simulink library "AUVLib"  (R2025b)
settings: Solver=VariableStepAuto  StartTime=0.0  StopTime=10.0  RelTol=1e-3
undefined symbols (not defined in the file): AUV, waterDensity
libraries: asbAUVlib x2, matrix_library x1, aerolibadyn x1, aerolibasang x1
settings Model: Creator=abshanka  LastModifiedBy=ubuntu

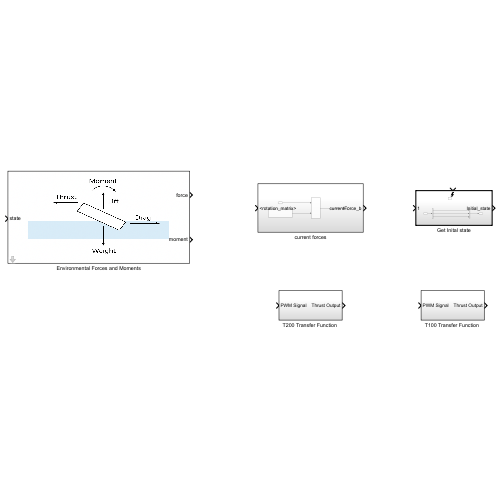
[thumbnail: Simulink's stored preview of the top-level diagram]
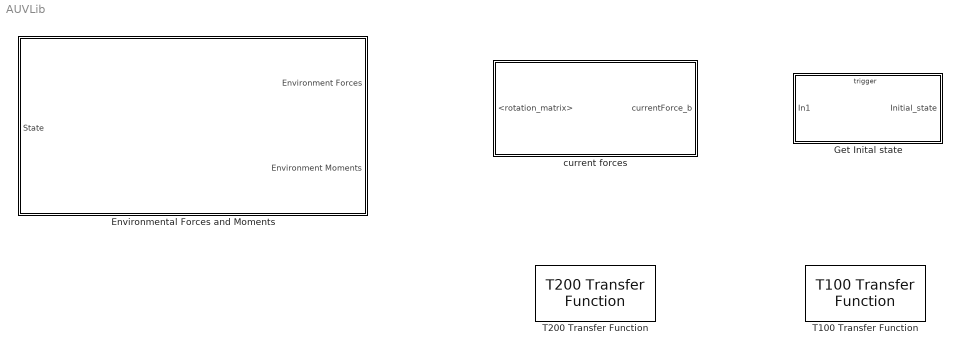
== system AUVLib ==
  Environmental Forces and Moments : Subsystem  mask{V=0.2056, h=AUV.Body.hulldiameter, mass=AUV.Body.mass, CoB=[0; 0; 0], Hy=Simple, ang_coeff=diag([ 10, 80,  82]), quad_coeff=diag([ 5,  32,  680]), lin_coeff=diag([ 3,  22,  220]), ang_coeff_c=diag([ 10, 80,  82]), alphaR=0, betaR=0, CX=0, CY=0, CZ=0, CMK=0, CMM=0, CMN=0, inputAxes=Body, cbar=1, b=1, S=1}
      mask prompts: V "Volume of AUV (m^3)"; h "Heigh (or diameter) of AUV (m)"; mass "Mass of AUV (kg)"; CoB "CoB (relative to CoM)"; Hy "Choose Hydrodynamics Simulation"; ang_coeff "Angular Damping coefficient"; quad_coeff "Quadratic drag coefficient"; lin_coeff "Linear drag coefficient"; ang_coeff_c "Angular Damping coefficient"; alphaR "Alpha Range"; betaR "Beta Range"; CX "Axial force coeff (CX)"; CY "Side force coeff (CY)"; CZ "Normal force coeff (CZ)"; CMK "Rolling moment coeff"; CMM "Pitching moment coeff"; CMN "Yawing moment coeff"; inputAxes "aeroblks:aeroblkadyn:blockAerodynamicForcesandMomentsParamInputaxes"; cbar "Length (m)"; b "Span (m)"; S "Ref Area (m^2)"
      mask TypeOptions V: Hydrostatics/volume displaced (m^3)/Value
      mask TypeOptions h: Hydrostatics/height/Value
      mask TypeOptions mass: Hydrostatics/Mass (Kg)/Value
      mask TypeOptions CoB: Hydrostatics/CoB (relative to CoM)(m)/Value
      mask TypeOptions inputAxes:
      | Variant Subsystem/Hydrodynamics_complex/Aerodynamic
      | Forces and Moments /inputAxes
      mask TypeOptions cbar:
      | Variant Subsystem/Hydrodynamics_complex/Aerodynamic
      | Forces and Moments /cbar
      mask TypeOptions b:
      | Variant Subsystem/Hydrodynamics_complex/Aerodynamic
      | Forces and Moments /b
      mask TypeOptions S:
      | Variant Subsystem/Hydrodynamics_complex/Aerodynamic
      | Forces and Moments /S
      mask DialogControl AUV_general Prompt: AUV Parameters (General)
      mask DialogControl AUV_hydro Prompt: AUV Hydrodynamics
      mask DialogControl Container5 Prompt: Simple Hydrodynamic Coeffs
      mask DialogControl Container6 Prompt: Complex Hydroynamics Coeffs
      mask DialogControl inputAxes Prompt: Input axes:
      mask Display:
      | image('force_moment.png');
      | port_label('output', 1, 'force');
      | port_label('output', 2, 'moment');
      | port_label('input', 1, 'state');
  Get Inital state : Subsystem
  "T100 Transfer Function " : asbAUVlib/T100 Transfer Function  SystemSampleTime=-1  VariantActivationTime=update diagram  EmptyChoice=off  PassThrough=off  PassThroughVariantControl=(default)  EmptyChoiceVariantControl=(default)  AllowFlexibleInterface=on  Latency=0  AutoFrameSizeCalculation=off
  "T200 Transfer Function " : asbAUVlib/T200 Transfer Function  SystemSampleTime=-1  VariantActivationTime=update diagram  EmptyChoice=off  PassThrough=off  PassThroughVariantControl=(default)  EmptyChoiceVariantControl=(default)  AllowFlexibleInterface=on  Latency=0  AutoFrameSizeCalculation=off
  current forces : Subsystem

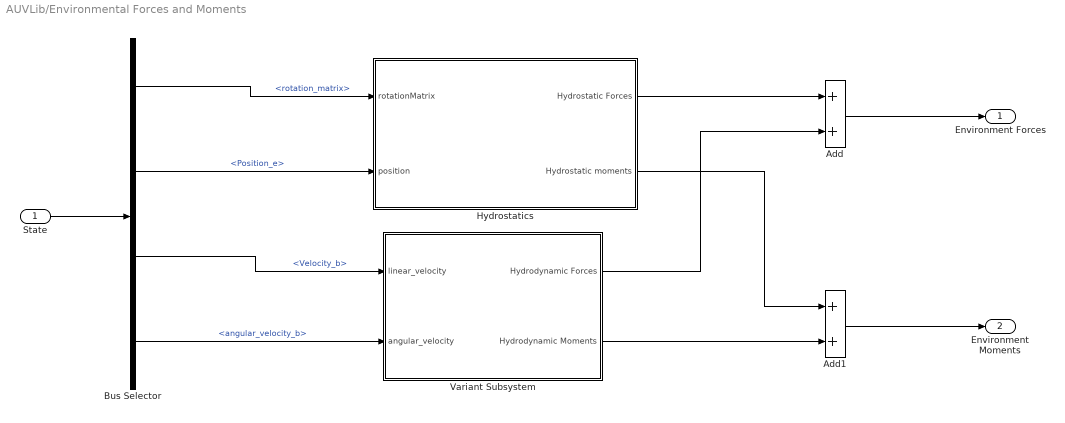
== system AUVLib/Environmental Forces and Moments ==
  State : Inport
  Add : Sum
  Add1 : Sum
  Bus Selector : BusSelector  OutputSignals=rotation_matrix,Position_e,Velocity_b,angular_velocity_b
  Hydrostatics : Subsystem
  Variant Subsystem : Subsystem  Variant=on
  Environment Forces : Outport
  Environment Moments : Outport  Port=2
  wires:
  Add1/1 -> Environment Moments/1
  Hydrostatics/2(Hydrostatic moments) -> Add1/1
  Add/1 -> Environment Forces/1
  State/1 -> Bus Selector/1
  Bus Selector/1 -> Hydrostatics/1(rotationMatrix)  "<rotation_matrix>"
  Bus Selector/2 -> Hydrostatics/2(position)  "<Position_e>"
  Hydrostatics/1(Hydrostatic Forces) -> Add/1
  Bus Selector/4 -> Variant Subsystem/2(angular_velocity)  "<angular_velocity_b>"
  Bus Selector/3 -> Variant Subsystem/1(linear_velocity)  "<Velocity_b>"
  Variant Subsystem/1(Hydrodynamic Forces) -> Add/2
  Variant Subsystem/2(Hydrodynamic Moments) -> Add1/2

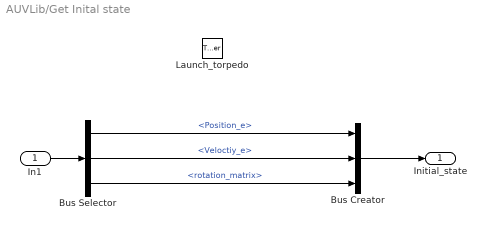
== system AUVLib/Get Inital state ==
  In1 : Inport
  Launch_torpedo : TriggerPort  VariantControl=(inherit)  PortDimensions=1
  Bus Creator : BusCreator  Inputs=3
  Bus Selector : BusSelector  OutputSignals=Position_e,Veloctiy_e,rotation_matrix
  Initial_state : Outport
  wires:
  Bus Selector/1 -> Bus Creator/1  "<Position_e>"
  Bus Selector/3 -> Bus Creator/3  "<rotation_matrix>"
  Bus Selector/2 -> Bus Creator/2  "<Veloctiy_e>"
  Bus Creator/1 -> Initial_state/1
  In1/1 -> Bus Selector/1

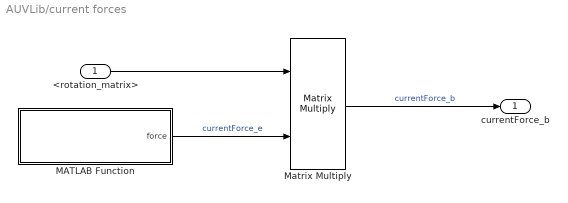
== system AUVLib/current forces ==
  <rotation_matrix> : Inport
  MATLAB Function : MATLAB Function  TreatAsAtomicUnit=on
  Matrix Multiply : Product  Multiplication=Matrix(*)
  currentForce_b : Outport
  wires:
  MATLAB Function/1(force) -> Matrix Multiply/2  "currentForce_e"
  Matrix Multiply/1 -> currentForce_b/1  "currentForce_b"
  <rotation_matrix>/1 -> Matrix Multiply/1

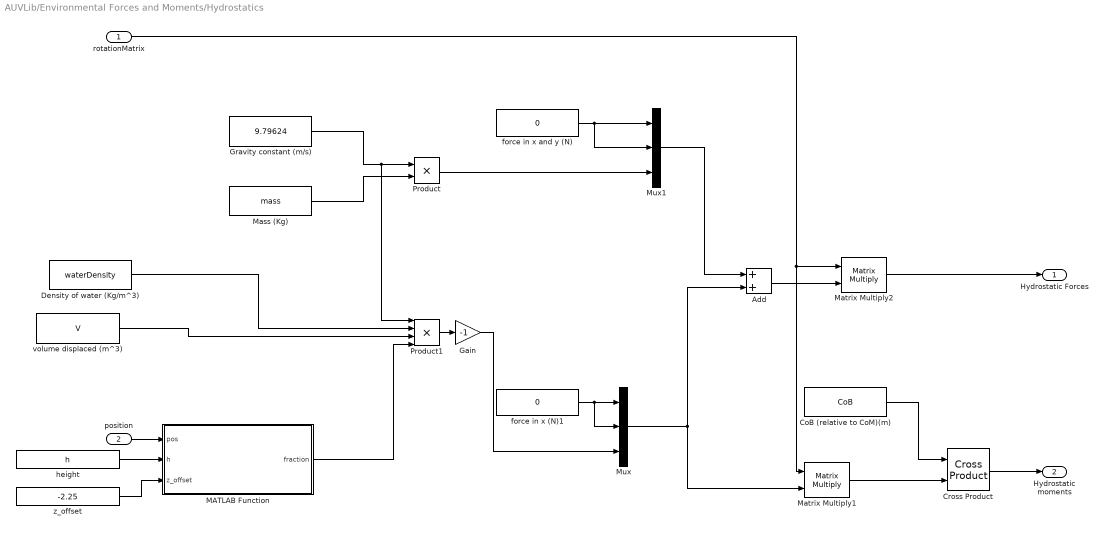
== system AUVLib/Environmental Forces and Moments/Hydrostatics ==
  rotationMatrix : Inport
  position : Inport  Port=2
  Add : Sum
  CoB (relative to CoM)(m) : Constant  Value=CoB
  Cross Product : matrix_library/Cross Product
  Density of water (Kg/m^3) : Constant  Value=waterDensity
  Gain : Gain  Gain=-1
  Gravity constant (m/s) : Constant  Value=9.79624
  MATLAB Function : MATLAB Function  TreatAsAtomicUnit=on
  Mass (Kg) : Constant  Value=mass
  Matrix Multiply1 : Product  Multiplication=Matrix(*)
  Matrix Multiply2 : Product  Multiplication=Matrix(*)
  Mux : Mux  Inputs=3
  Mux1 : Mux  Inputs=3
  Product : Product
  Product1 : Product  Inputs=4
  force in x (N)1 : Constant  Value=0
  force in x and y (N) : Constant  Value=0
  height : Constant  Value=h
  volume displaced (m^3) : Constant  Value=V
  z_offset : Constant  Value=-2.25
  Hydrostatic Forces : Outport
  Hydrostatic moments : Outport  Port=2
  wires:
  Gravity constant (m/s)/1 -> Product1/1, Product/1
  Mux/1 -> Add/2, Matrix Multiply1/2
  CoB (relative to CoM)(m)/1 -> Cross Product/1
  volume displaced (m^3)/1 -> Product1/3
  rotationMatrix/1 -> Matrix Multiply2/1, Matrix Multiply1/1
  MATLAB Function/1(fraction) -> Product1/4
  force in x (N)1/1 -> Mux/2, Mux/1
  Mux1/1 -> Add/1
  Product/1 -> Mux1/3
  Product1/1 -> Gain/1
  Add/1 -> Matrix Multiply2/2
  force in x and y (N)/1 -> Mux1/2, Mux1/1
  Density of water (Kg/m^3)/1 -> Product1/2
  Mass (Kg)/1 -> Product/2
  Cross Product/1 -> Hydrostatic moments/1
  Matrix Multiply1/1 -> Cross Product/2
  Matrix Multiply2/1 -> Hydrostatic Forces/1
  position/1 -> MATLAB Function/1(pos)
  height/1 -> MATLAB Function/2(h)
  Gain/1 -> Mux/3
  z_offset/1 -> MATLAB Function/3(z_offset)

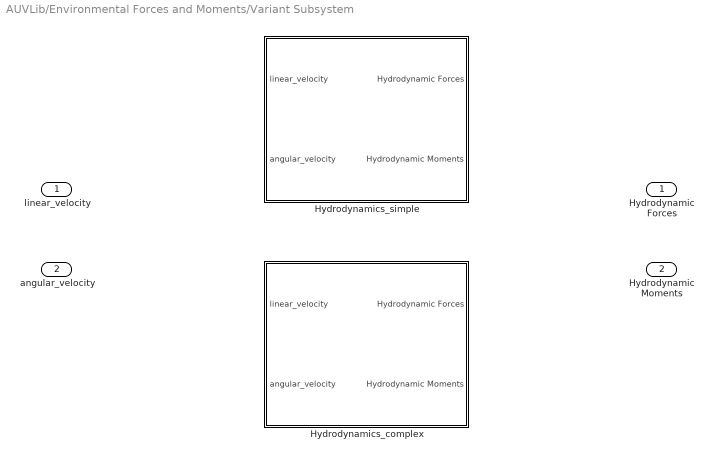
== system AUVLib/Environmental Forces and Moments/Variant Subsystem ==
  linear_velocity : Inport
  angular_velocity : Inport  Port=2
  Hydrodynamics_complex : Subsystem  VariantControl=Hy == 2
  Hydrodynamics_simple : Subsystem  VariantControl=Hy == 1
  Hydrodynamic Forces : Outport
  Hydrodynamic Moments : Outport  Port=2

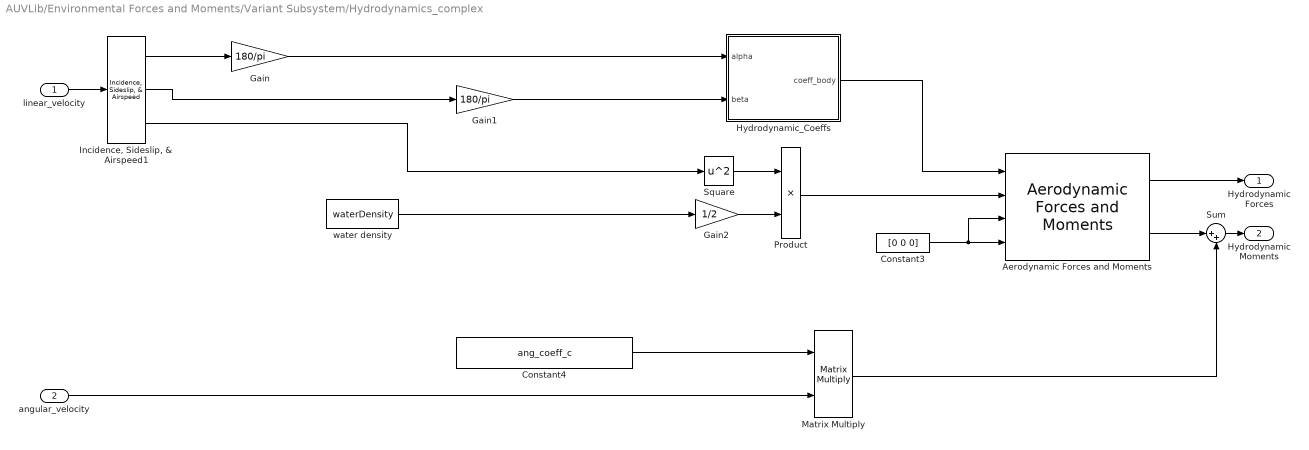
== system AUVLib/Environmental Forces and Moments/Variant Subsystem/Hydrodynamics_complex ==
  linear_velocity : Inport
  angular_velocity : Inport  Port=2
  "Aerodynamic Forces and Moments " : aerolibadyn/Aerodynamic Forces and Moments   inputAxes=Body  outputForceAxes=Body  outputMomentAxes=Body  S=S  b=b  cbar=cbar
  Constant3 : Constant  Value=[0 0 0]
  Constant4 : Constant  Value=ang_coeff_c
  Gain : Gain  Gain=180/pi
  Gain1 : Gain  Gain=180/pi
  Gain2 : Gain  Gain=1/2
  Hydrodynamic_Coeffs : Subsystem
  "Incidence, Sideslip, & Airspeed1" : aerolibasang/Incidence, Sideslip, & Airspeed
  Matrix Multiply : Product  Multiplication=Matrix(*)
  Product : Product
  Square : Math  Operator=square
  Sum : Sum  Inputs=|++
  water density : Constant  Value=waterDensity
  Hydrodynamic Forces : Outport
  Hydrodynamic Moments : Outport  Port=2
  wires:
  linear_velocity/1 -> "Incidence, Sideslip, & Airspeed1"/1
  Sum/1 -> Hydrodynamic Moments/1
  Matrix Multiply/1 -> Sum/2
  Product/1 -> "Aerodynamic Forces and Moments "/2
  "Aerodynamic Forces and Moments "/1 -> Hydrodynamic Forces/1
  angular_velocity/1 -> Matrix Multiply/2
  water density/1 -> Gain2/1
  "Incidence, Sideslip, & Airspeed1"/2 -> Gain1/1
  "Incidence, Sideslip, & Airspeed1"/3 -> Square/1
  "Incidence, Sideslip, & Airspeed1"/1 -> Gain/1
  Hydrodynamic_Coeffs/1(coeff_body) -> "Aerodynamic Forces and Moments "/1
  Constant4/1 -> Matrix Multiply/1
  Gain2/1 -> Product/2
  Gain/1 -> Hydrodynamic_Coeffs/1(alpha)
  Square/1 -> Product/1
  Gain1/1 -> Hydrodynamic_Coeffs/2(beta)
  Constant3/1 -> "Aerodynamic Forces and Moments "/4, "Aerodynamic Forces and Moments "/3
  "Aerodynamic Forces and Moments "/2 -> Sum/1

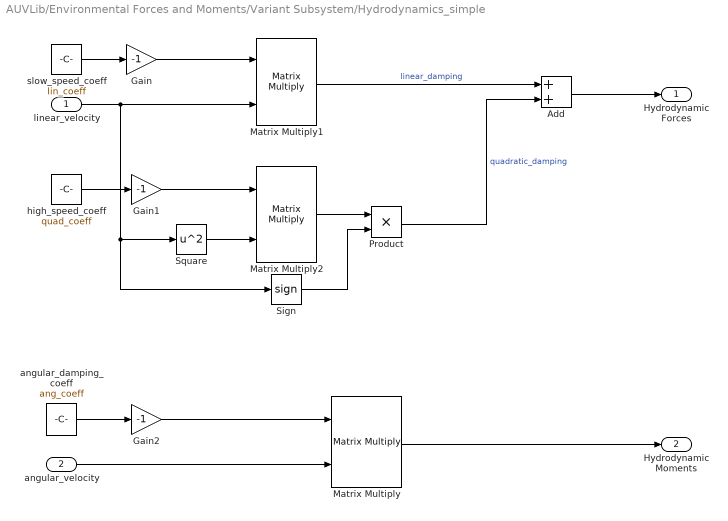
== system AUVLib/Environmental Forces and Moments/Variant Subsystem/Hydrodynamics_simple ==
  linear_velocity : Inport
  angular_velocity : Inport  Port=2
  Add : Sum
  Gain : Gain  Gain=-1
  Gain1 : Gain  Gain=-1
  Gain2 : Gain  Gain=-1
  Matrix Multiply : Product  Multiplication=Matrix(*)
  Matrix Multiply1 : Product  Multiplication=Matrix(*)
  Matrix Multiply2 : Product  Multiplication=Matrix(*)
  Product : Product
  Sign : Signum
  Square : Math  Operator=square
  angular_damping_coeff : Constant  Value=ang_coeff
  high_speed_coeff : Constant  Value=quad_coeff
  slow_speed_coeff : Constant  Value=lin_coeff
  Hydrodynamic Forces : Outport
  Hydrodynamic Moments : Outport  Port=2
  wires:
  Matrix Multiply/1 -> Hydrodynamic Moments/1
  angular_velocity/1 -> Matrix Multiply/2
  Add/1 -> Hydrodynamic Forces/1
  high_speed_coeff/1 -> Gain1/1
  Sign/1 -> Product/2
  Matrix Multiply1/1 -> Add/1  "linear_damping"
  Matrix Multiply2/1 -> Product/1
  slow_speed_coeff/1 -> Gain/1
  Square/1 -> Matrix Multiply2/2
  Product/1 -> Add/2  "quadratic_damping"
  angular_damping_coeff/1 -> Gain2/1
  linear_velocity/1 -> Matrix Multiply1/2, Square/1, Sign/1
  Gain/1 -> Matrix Multiply1/1
  Gain1/1 -> Matrix Multiply2/1
  Gain2/1 -> Matrix Multiply/1

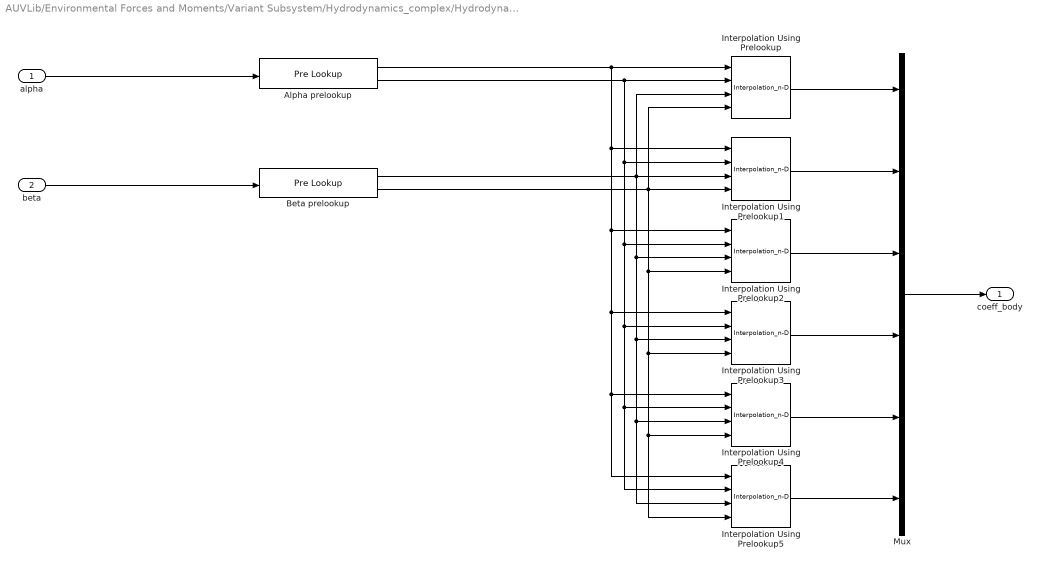
== system AUVLib/Environmental Forces and Moments/Variant Subsystem/Hydrodynamics_complex/Hydrodynamic_Coeffs ==
  alpha : Inport
  beta : Inport  Port=2
  Alpha prelookup : PreLookup  BreakpointsData=alphaR  ExtrapMethod=Linear
  Beta prelookup : PreLookup  BreakpointsData=betaR  ExtrapMethod=Linear
  Interpolation Using Prelookup : Interpolation_n-D  Table=CX'  InternalRulePriority=Speed
  Interpolation Using Prelookup1 : Interpolation_n-D  Table=CY'  InternalRulePriority=Speed
  Interpolation Using Prelookup2 : Interpolation_n-D  Table=CZ'  InternalRulePriority=Speed
  Interpolation Using Prelookup3 : Interpolation_n-D  Table=CMK'  InternalRulePriority=Speed
  Interpolation Using Prelookup4 : Interpolation_n-D  Table=CMM'  InternalRulePriority=Speed
  Interpolation Using Prelookup5 : Interpolation_n-D  Table=CMN'  InternalRulePriority=Speed
  Mux : Mux  Inputs=6
  coeff_body : Outport
  wires:
  Mux/1 -> coeff_body/1
  Interpolation Using Prelookup5/1 -> Mux/6
  Interpolation Using Prelookup3/1 -> Mux/4
  Interpolation Using Prelookup4/1 -> Mux/5
  Interpolation Using Prelookup1/1 -> Mux/2
  Interpolation Using Prelookup2/1 -> Mux/3
  Interpolation Using Prelookup/1 -> Mux/1
  beta/1 -> Beta prelookup/1
  alpha/1 -> Alpha prelookup/1
  Beta prelookup/2 -> Interpolation Using Prelookup1/4, Interpolation Using Prelookup5/4, Interpolation Using Prelookup4/4, Interpolation Using Prelookup3/4, Interpolation Using Prelookup2/4, Interpolation Using Prelookup/4
  Beta prelookup/1 -> Interpolation Using Prelookup1/3, Interpolation Using Prelookup5/3, Interpolation Using Prelookup4/3, Interpolation Using Prelookup3/3, Interpolation Using Prelookup2/3, Interpolation Using Prelookup/3
  Alpha prelookup/1 -> Interpolation Using Prelookup/1, Interpolation Using Prelookup5/1, Interpolation Using Prelookup4/1, Interpolation Using Prelookup3/1, Interpolation Using Prelookup2/1, Interpolation Using Prelookup1/1
  Alpha prelookup/2 -> Interpolation Using Prelookup/2, Interpolation Using Prelookup5/2, Interpolation Using Prelookup4/2, Interpolation Using Prelookup3/2, Interpolation Using Prelookup2/2, Interpolation Using Prelookup1/2

== matlab function AUVLib/Environmental Forces and Moments/Hydrostatics/MATLAB Function ==
  data: pos input; fraction output; h input; z_offset input
function fraction = getFractionSubmerged(pos, h, z_offset)

if pos(3) >= (h/2 + z_offset)
    fraction = 1;
elseif pos(3) <= (-h/2 + z_offset)
    fraction = 0;
else
    fraction = (pos(3) - z_offset)/h + 0.5;
end

== matlab function AUVLib/current forces/MATLAB Function ==
  data: force output
function force = getCurrentForce()
    
    force = zeros([3,1]);
    force_dir = -pi + rand(1)*(2*pi);
    force_min = 0.15;
    force_max = 0.3;
    force_val = force_min + rand(1)*(force_max - force_min);

    force(1,1) = force_val*cos(force_dir);
    force(2,1) = force_val*sin(force_dir);
